simulink library "Weather_Simple_Model"  (Simulink 8.2)
settings: Solver=ode45  StartTime=0.0  StopTime=10.0  RelTol=1e-3
libraries: carnot x4, simulink x1
settings Model: Creator=lena.frank  LastModifiedBy=drhf

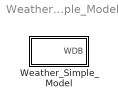
== system Weather_Simple_Model ==
  Weather_Simple_Model : Subsystem  mask(Weather Simple Model){lat=60, Ibn=900, Idg=100, tamb=5, deltaTsky=-6, rh=50, precip=10e-3/24/3600           % 10 mm in 24 h, cloud=0.125, p=1013e2, vw=1, wdir=270}
      mask prompts: lat "Latitude in degree (north positve)"; Ibn "Maximum beam radiation on normal surface in W/m²"; Idg "Maximum diffuse radiation on horizontal surface in W/m²"; tamb "Ambient temperature in °C"; deltaTsky "Offset for sky temperature in K (usually -6K)"; rh "Relative humidity in %"; precip "Rainfall (precipitation) in m/s"; cloud "Cloud index in (0..1)"; p "Air pressure in Pa"; vw "Wind speed in m/s"; wdir "Wind direction in ° (0° = North, 90° = East)"
      mask help:
      | Create a simple, mostly constant weather data bus (WDB).
      | The solar radiation corresponds to clear sky conditions.
      mask Help: web(fullfile(path_carnot('help'),'Weather_Simple_Model.html'),'-helpbrowser')

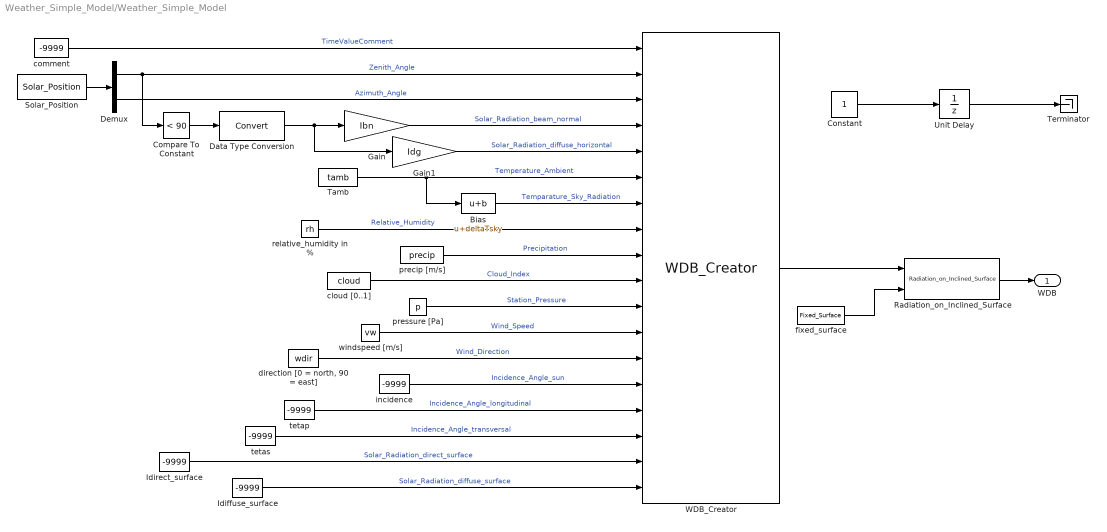
== system Weather_Simple_Model/Weather_Simple_Model ==
  Bias : Bias  Bias=deltaTsky
  Compare To Constant : simulink/Logic and Bit Operations/Compare To Constant  relop=<  const=90  OutDataTypeStr=uint8
  Constant : Constant
  Data Type Conversion : DataTypeConversion
  Demux : Demux  Outputs=2
  Gain : Gain  Gain=Ibn
  Gain1 : Gain  Gain=Idg
  Idiffuse_surface : Constant  Value=-9999
  Idirect_surface : Constant  Value=-9999
  Radiation_on_Inclined_Surface : carnot/Weather/Radiation_on_Inclined_Surface  sky=Perez 1990  reflect=0.2
  Solar_Position : carnot/Basic/Weather_and_Sun/Solar_Position  lati=lat  longi=0  timezone=0
  Tamb : Constant  Value=tamb
  Terminator : Terminator
  Unit Delay : UnitDelay  SampleTime=3600
  WDB_Creator : carnot/Basic/Weather_and_Sun/WDB_Creator
  cloud [0..1] : Constant  Value=cloud
  comment : Constant  Value=-9999
  "direction [0 = north, 90 = east]" : Constant  Value=wdir
  fixed_surface : carnot/Weather/Fixed_Surface  colangle=0  colazi=0  colrot=0
  incidence : Constant  Value=-9999
  precip [m/s] : Constant  Value=precip
  pressure [Pa] : Constant  Value=p
  relative_humidity in % : Constant  Value=rh
  tetap : Constant  Value=-9999
  tetas : Constant  Value=-9999
  windspeed [m/s] : Constant  Value=vw
  WDB : Outport
  wires:
  WDB_Creator/1 -> Radiation_on_Inclined_Surface/1
  Radiation_on_Inclined_Surface/1 -> WDB/1
  fixed_surface/1 -> Radiation_on_Inclined_Surface/2
  Gain/1 -> WDB_Creator/4  "Solar_Radiation_beam_normal"
  Solar_Position/1 -> Demux/1
  comment/1 -> WDB_Creator/1  "TimeValueComment"
  Demux/1 -> WDB_Creator/2, Compare To Constant/1  "Zenith_Angle"
  Demux/2 -> WDB_Creator/3  "Azimuth_Angle"
  Compare To Constant/1 -> Data Type Conversion/1
  Gain1/1 -> WDB_Creator/5  "Solar_Radiation_diffuse_horizontal"
  Tamb/1 -> WDB_Creator/6, Bias/1  "Temperature_Ambient"
  Bias/1 -> WDB_Creator/7  "Temparature_Sky_Radiation"
  relative_humidity in %/1 -> WDB_Creator/8  "Relative_Humidity"
  precip [m/s]/1 -> WDB_Creator/9  "Precipitation"
  cloud [0..1]/1 -> WDB_Creator/10  "Cloud_Index"
  pressure [Pa]/1 -> WDB_Creator/11  "Station_Pressure"
  windspeed [m/s]/1 -> WDB_Creator/12  "Wind_Speed"
  "direction [0 = north, 90 = east]"/1 -> WDB_Creator/13  "Wind_Direction"
  incidence/1 -> WDB_Creator/14  "Incidence_Angle_sun"
  tetap/1 -> WDB_Creator/15  "Incidence_Angle_longitudinal"
  tetas/1 -> WDB_Creator/16  "Incidence_Angle_transversal"
  Idirect_surface/1 -> WDB_Creator/17  "Solar_Radiation_direct_surface"
  Idiffuse_surface/1 -> WDB_Creator/18  "Solar_Radiation_diffuse_surface"
  Data Type Conversion/1 -> Gain1/1, Gain/1
  Constant/1 -> Unit Delay/1
  Unit Delay/1 -> Terminator/1
